simulink model "Temps_Reponse"  (R2016b)
settings: Solver=VariableStepAuto  StartTime=0.0  StopTime=4.0  RelTol=1e-3
settings Model: Creator=pt_ptsi  LastModifiedBy=pt_ptsi

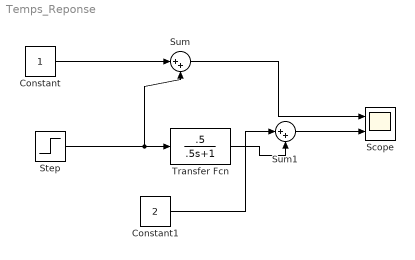
== system Temps_Reponse ==
  Constant : Constant
  Constant1 : Constant  Value=2
  Scope : Scope  NumInputPorts=2
  Step : Step  After=4  SampleTime=0
  Sum : Sum  Inputs=|++
  Sum1 : Sum  Inputs=|++
  Transfer Fcn : TransferFcn  Numerator=[.5]  Denominator=[.5 1]
  wires:
  Step/1 -> Sum/2, Transfer Fcn/1
  Constant/1 -> Sum/1
  Sum/1 -> Scope/1
  Transfer Fcn/1 -> Sum1/2
  Constant1/1 -> Sum1/1
  Sum1/1 -> Scope/2
